simulink model "SCCS_Integration_05"  (R2024a)
settings: Solver=ode3  StartTime=0.0  StopTime=20.0  FixedStep=0.01  RelTol=1e-3
settings Model: Creator=Kishore  LastModifiedBy=Kishore

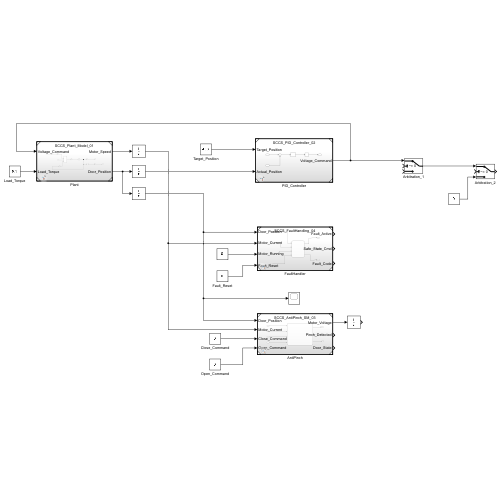
[thumbnail: Simulink's stored preview of the top-level diagram]
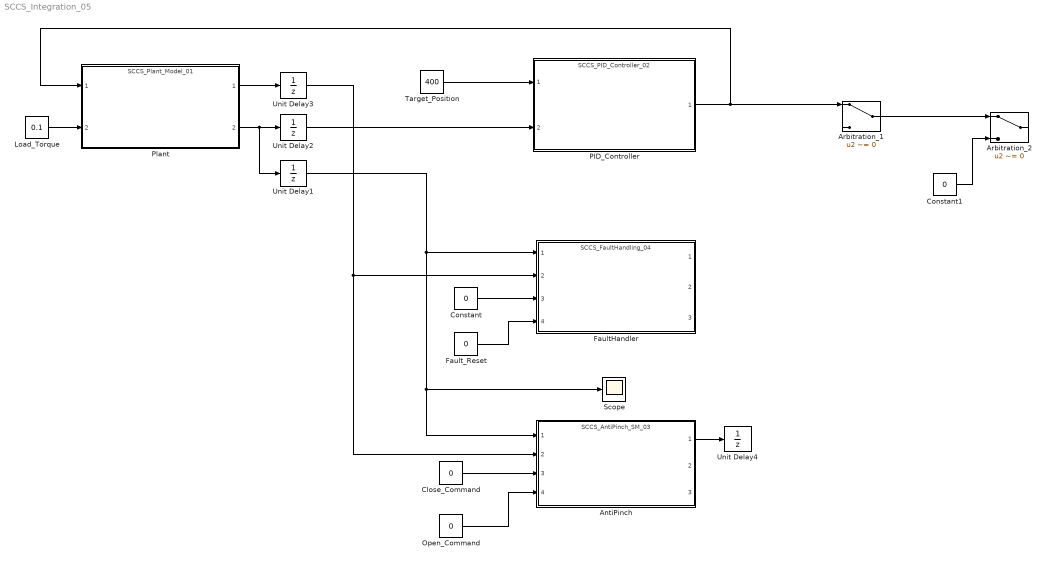
== system SCCS_Integration_05 ==
  AntiPinch : ModelReference  ModelNameDialog=SCCS_AntiPinch_SM_03.slx  SimulationMode=Normal  ModelReferenceVersion=1.14
  Arbitration_1 : Switch  Criteria=u2 ~= 0  SaturateOnIntegerOverflow=off  InputSameDT=off
  Arbitration_2 : Switch  Criteria=u2 ~= 0  SaturateOnIntegerOverflow=off  InputSameDT=off
  Close_Command : Constant  Value=0
  Constant : Constant  Value=0
  Constant1 : Constant  Value=0
  FaultHandler : ModelReference  ModelNameDialog=SCCS_FaultHandling_04.slx  SimulationMode=Normal  ModelReferenceVersion=1.12
  Fault_Reset : Constant  Value=0
  Load_Torque : Constant  Value=0.1
  Open_Command : Constant  Value=0
  PID_Controller : ModelReference  ModelNameDialog=SCCS_PID_Controller_02.slx  SimulationMode=Normal  ModelReferenceVersion=1.13
  Plant : ModelReference  ModelNameDialog=SCCS_Plant_Model_01.slx  SimulationMode=Normal  ModelReferenceVersion=1.15
  Scope : Scope
  Target_Position : Constant  Value=400
  Unit Delay{1..4} (4 alike) : UnitDelay  SampleTime=0.01  HasFrameUpgradeWarning=on
  wires:
  Target_Position/1 -> PID_Controller/1
  Load_Torque/1 -> Plant/2
  Close_Command/1 -> AntiPinch/3
  Open_Command/1 -> AntiPinch/4
  Fault_Reset/1 -> FaultHandler/4
  Constant/1 -> FaultHandler/3
  AntiPinch/1 -> Unit Delay4/1
  Constant1/1 -> Arbitration_2/3
  Plant/2 -> Unit Delay1/1, Unit Delay2/1
  Plant/1 -> Unit Delay3/1
  Unit Delay2/1 -> PID_Controller/2
  Unit Delay1/1 -> Scope/1, AntiPinch/1, FaultHandler/1
  Unit Delay3/1 -> AntiPinch/2, FaultHandler/2
  PID_Controller/1 -> Arbitration_1/1, Plant/1
  Arbitration_1/1 -> Arbitration_2/1
